simulink model "kurtosis"  (R2012b)
settings: Solver=ode45  StartTime=0.0  StopTime=3171  RelTol=1e-3
libraries: xbsIndex_r4 x3174, casper_library_flow_control x64, casper_library_misc x1, simulink_xsg_bridge x1
(part 2 of 24)

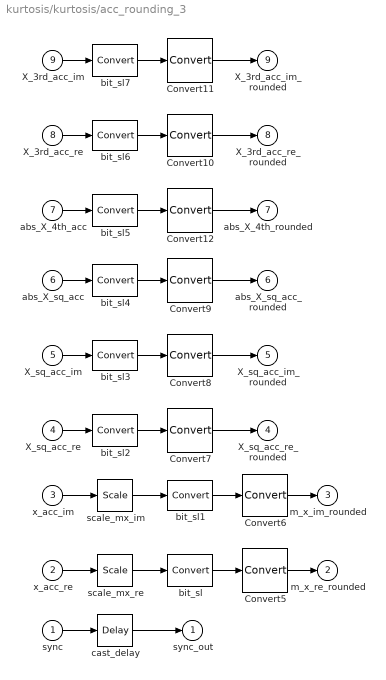
== system kurtosis/kurtosis/acc_rounding_3 ==
  sync : Inport
  x_acc_re : Inport  Port=2
  x_acc_im : Inport  Port=3
  X_sq_acc_re : Inport  Port=4
  X_sq_acc_im : Inport  Port=5
  abs_X_sq_acc : Inport  Port=6
  abs_X_4th_acc : Inport  Port=7
  X_3rd_acc_re : Inport  Port=8
  X_3rd_acc_im : Inport  Port=9
  Convert{7..11} (5 alike) : xbsIndex_r4/Convert  gui_display_data_type=Fixed-point  arith_type="Signed  (2's comp)"  n_bits=35  bin_pt=22  float_type=Single  exp_bits=8  fraction_bits=24  quantization="Round  (unbiased: +/- Inf)"  overflow=Saturate  en=off  latency=5  dbl_ovrd=off  pipeline=off  block_type=convert
  Convert12 : xbsIndex_r4/Convert  gui_display_data_type=Fixed-point  arith_type="Signed  (2's comp)"  n_bits=84  bin_pt=68  float_type=Single  exp_bits=8  fraction_bits=24  quantization="Round  (unbiased: +/- Inf)"  overflow=Saturate  en=off  latency=5  dbl_ovrd=off  pipeline=off  block_type=convert
  Convert5 : xbsIndex_r4/Convert  gui_display_data_type=Fixed-point  arith_type="Signed  (2's comp)"  n_bits=25  bin_pt=24  float_type=Single  exp_bits=8  fraction_bits=24  quantization="Round  (unbiased: +/- Inf)"  overflow=Saturate  en=off  latency=5  dbl_ovrd=off  pipeline=off  block_type=convert
  Convert6 : xbsIndex_r4/Convert  gui_display_data_type=Fixed-point  arith_type="Signed  (2's comp)"  n_bits=25  bin_pt=24  float_type=Single  exp_bits=8  fraction_bits=24  quantization="Round  (unbiased: +/- Inf)"  overflow=Saturate  en=off  latency=5  dbl_ovrd=off  pipeline=off  block_type=convert
  bit_sl : xbsIndex_r4/Convert  gui_display_data_type=Fixed-point  arith_type="Signed  (2's comp)"  n_bits=28  bin_pt=27  float_type=Single  exp_bits=8  fraction_bits=24  quantization=Truncate  overflow=Wrap  en=off  latency=0  dbl_ovrd=off  pipeline=off  block_type=convert
  bit_sl1 : xbsIndex_r4/Convert  gui_display_data_type=Fixed-point  arith_type="Signed  (2's comp)"  n_bits=28  bin_pt=27  float_type=Single  exp_bits=8  fraction_bits=24  quantization=Truncate  overflow=Wrap  en=off  latency=0  dbl_ovrd=off  pipeline=off  block_type=convert
  bit_sl2 : xbsIndex_r4/Convert  gui_display_data_type=Fixed-point  arith_type="Signed  (2's comp)"  n_bits=47  bin_pt=34  float_type=Single  exp_bits=8  fraction_bits=24  quantization=Truncate  overflow=Wrap  en=off  latency=0  dbl_ovrd=off  pipeline=off  block_type=convert
  bit_sl3 : xbsIndex_r4/Convert  gui_display_data_type=Fixed-point  arith_type="Signed  (2's comp)"  n_bits=47  bin_pt=34  float_type=Single  exp_bits=8  fraction_bits=24  quantization=Truncate  overflow=Wrap  en=off  latency=0  dbl_ovrd=off  pipeline=off  block_type=convert
  bit_sl4 : xbsIndex_r4/Convert  gui_display_data_type=Fixed-point  arith_type="Signed  (2's comp)"  n_bits=47  bin_pt=34  float_type=Single  exp_bits=8  fraction_bits=24  quantization=Truncate  overflow=Wrap  en=off  latency=0  dbl_ovrd=off  pipeline=off  block_type=convert
  bit_sl5 : xbsIndex_r4/Convert  gui_display_data_type=Fixed-point  arith_type="Signed  (2's comp)"  n_bits=84  bin_pt=68  float_type=Single  exp_bits=8  fraction_bits=24  quantization=Truncate  overflow=Wrap  en=off  latency=0  dbl_ovrd=off  pipeline=off  block_type=convert
  bit_sl6 : xbsIndex_r4/Convert  gui_display_data_type=Fixed-point  arith_type="Signed  (2's comp)"  n_bits=64  bin_pt=51  float_type=Single  exp_bits=8  fraction_bits=24  quantization=Truncate  overflow=Wrap  en=off  latency=0  dbl_ovrd=off  pipeline=off  block_type=convert
  bit_sl7 : xbsIndex_r4/Convert  gui_display_data_type=Fixed-point  arith_type="Signed  (2's comp)"  n_bits=64  bin_pt=51  float_type=Single  exp_bits=8  fraction_bits=24  quantization=Truncate  overflow=Wrap  en=off  latency=0  dbl_ovrd=off  pipeline=off  block_type=convert
  cast_delay : xbsIndex_r4/Delay  rst=off  infoeditControl=Selection of Reset will increase slice count due to use of real FFs and instead of SRLs  en=off  latency=5  dbl_ovrd=off  reg_retiming=off  block_type=delay
  scale_mx_im : xbsIndex_r4/Scale  scale_factor=-10  dbl_ovrd=off  block_type=scale
  scale_mx_re : xbsIndex_r4/Scale  scale_factor=-10  dbl_ovrd=off  block_type=scale
  sync_out : Outport
  m_x_re_rounded : Outport  Port=2
  m_x_im_rounded : Outport  Port=3
  X_sq_acc_re_rounded : Outport  Port=4
  X_sq_acc_im_rounded : Outport  Port=5
  abs_X_sq_acc_rounded : Outport  Port=6
  abs_X_4th_rounded : Outport  Port=7
  X_3rd_acc_re_rounded : Outport  Port=8
  X_3rd_acc_im_rounded : Outport  Port=9
  wires:
  cast_delay/1 -> sync_out/1
  sync/1 -> cast_delay/1
  Convert11/1 -> X_3rd_acc_im_rounded/1
  bit_sl7/1 -> Convert11/1
  Convert10/1 -> X_3rd_acc_re_rounded/1
  bit_sl6/1 -> Convert10/1
  Convert12/1 -> abs_X_4th_rounded/1
  bit_sl5/1 -> Convert12/1
  Convert9/1 -> abs_X_sq_acc_rounded/1
  bit_sl4/1 -> Convert9/1
  Convert8/1 -> X_sq_acc_im_rounded/1
  bit_sl3/1 -> Convert8/1
  Convert7/1 -> X_sq_acc_re_rounded/1
  bit_sl2/1 -> Convert7/1
  Convert6/1 -> m_x_im_rounded/1
  bit_sl1/1 -> Convert6/1
  Convert5/1 -> m_x_re_rounded/1
  bit_sl/1 -> Convert5/1
  X_3rd_acc_im/1 -> bit_sl7/1
  X_3rd_acc_re/1 -> bit_sl6/1
  abs_X_4th_acc/1 -> bit_sl5/1
  abs_X_sq_acc/1 -> bit_sl4/1
  X_sq_acc_im/1 -> bit_sl3/1
  X_sq_acc_re/1 -> bit_sl2/1
  scale_mx_im/1 -> bit_sl1/1
  scale_mx_re/1 -> bit_sl/1
  x_acc_im/1 -> scale_mx_im/1
  x_acc_re/1 -> scale_mx_re/1

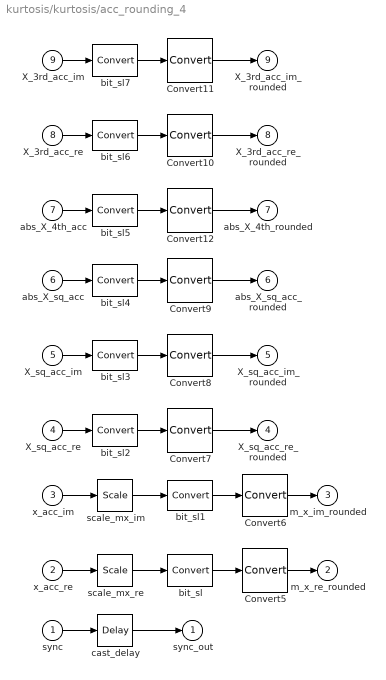
== system kurtosis/kurtosis/acc_rounding_4 ==
  sync : Inport
  x_acc_re : Inport  Port=2
  x_acc_im : Inport  Port=3
  X_sq_acc_re : Inport  Port=4
  X_sq_acc_im : Inport  Port=5
  abs_X_sq_acc : Inport  Port=6
  abs_X_4th_acc : Inport  Port=7
  X_3rd_acc_re : Inport  Port=8
  X_3rd_acc_im : Inport  Port=9
  Convert{7..11} (5 alike) : xbsIndex_r4/Convert  gui_display_data_type=Fixed-point  arith_type="Signed  (2's comp)"  n_bits=35  bin_pt=22  float_type=Single  exp_bits=8  fraction_bits=24  quantization="Round  (unbiased: +/- Inf)"  overflow=Saturate  en=off  latency=5  dbl_ovrd=off  pipeline=off  block_type=convert
  Convert12 : xbsIndex_r4/Convert  gui_display_data_type=Fixed-point  arith_type="Signed  (2's comp)"  n_bits=84  bin_pt=68  float_type=Single  exp_bits=8  fraction_bits=24  quantization="Round  (unbiased: +/- Inf)"  overflow=Saturate  en=off  latency=5  dbl_ovrd=off  pipeline=off  block_type=convert
  Convert5 : xbsIndex_r4/Convert  gui_display_data_type=Fixed-point  arith_type="Signed  (2's comp)"  n_bits=25  bin_pt=24  float_type=Single  exp_bits=8  fraction_bits=24  quantization="Round  (unbiased: +/- Inf)"  overflow=Saturate  en=off  latency=5  dbl_ovrd=off  pipeline=off  block_type=convert
  Convert6 : xbsIndex_r4/Convert  gui_display_data_type=Fixed-point  arith_type="Signed  (2's comp)"  n_bits=25  bin_pt=24  float_type=Single  exp_bits=8  fraction_bits=24  quantization="Round  (unbiased: +/- Inf)"  overflow=Saturate  en=off  latency=5  dbl_ovrd=off  pipeline=off  block_type=convert
  bit_sl : xbsIndex_r4/Convert  gui_display_data_type=Fixed-point  arith_type="Signed  (2's comp)"  n_bits=28  bin_pt=27  float_type=Single  exp_bits=8  fraction_bits=24  quantization=Truncate  overflow=Wrap  en=off  latency=0  dbl_ovrd=off  pipeline=off  block_type=convert
  bit_sl1 : xbsIndex_r4/Convert  gui_display_data_type=Fixed-point  arith_type="Signed  (2's comp)"  n_bits=28  bin_pt=27  float_type=Single  exp_bits=8  fraction_bits=24  quantization=Truncate  overflow=Wrap  en=off  latency=0  dbl_ovrd=off  pipeline=off  block_type=convert
  bit_sl2 : xbsIndex_r4/Convert  gui_display_data_type=Fixed-point  arith_type="Signed  (2's comp)"  n_bits=47  bin_pt=34  float_type=Single  exp_bits=8  fraction_bits=24  quantization=Truncate  overflow=Wrap  en=off  latency=0  dbl_ovrd=off  pipeline=off  block_type=convert
  bit_sl3 : xbsIndex_r4/Convert  gui_display_data_type=Fixed-point  arith_type="Signed  (2's comp)"  n_bits=47  bin_pt=34  float_type=Single  exp_bits=8  fraction_bits=24  quantization=Truncate  overflow=Wrap  en=off  latency=0  dbl_ovrd=off  pipeline=off  block_type=convert
  bit_sl4 : xbsIndex_r4/Convert  gui_display_data_type=Fixed-point  arith_type="Signed  (2's comp)"  n_bits=47  bin_pt=34  float_type=Single  exp_bits=8  fraction_bits=24  quantization=Truncate  overflow=Wrap  en=off  latency=0  dbl_ovrd=off  pipeline=off  block_type=convert
  bit_sl5 : xbsIndex_r4/Convert  gui_display_data_type=Fixed-point  arith_type="Signed  (2's comp)"  n_bits=84  bin_pt=68  float_type=Single  exp_bits=8  fraction_bits=24  quantization=Truncate  overflow=Wrap  en=off  latency=0  dbl_ovrd=off  pipeline=off  block_type=convert
  bit_sl6 : xbsIndex_r4/Convert  gui_display_data_type=Fixed-point  arith_type="Signed  (2's comp)"  n_bits=64  bin_pt=51  float_type=Single  exp_bits=8  fraction_bits=24  quantization=Truncate  overflow=Wrap  en=off  latency=0  dbl_ovrd=off  pipeline=off  block_type=convert
  bit_sl7 : xbsIndex_r4/Convert  gui_display_data_type=Fixed-point  arith_type="Signed  (2's comp)"  n_bits=64  bin_pt=51  float_type=Single  exp_bits=8  fraction_bits=24  quantization=Truncate  overflow=Wrap  en=off  latency=0  dbl_ovrd=off  pipeline=off  block_type=convert
  cast_delay : xbsIndex_r4/Delay  rst=off  infoeditControl=Selection of Reset will increase slice count due to use of real FFs and instead of SRLs  en=off  latency=5  dbl_ovrd=off  reg_retiming=off  block_type=delay
  scale_mx_im : xbsIndex_r4/Scale  scale_factor=-10  dbl_ovrd=off  block_type=scale
  scale_mx_re : xbsIndex_r4/Scale  scale_factor=-10  dbl_ovrd=off  block_type=scale
  sync_out : Outport
  m_x_re_rounded : Outport  Port=2
  m_x_im_rounded : Outport  Port=3
  X_sq_acc_re_rounded : Outport  Port=4
  X_sq_acc_im_rounded : Outport  Port=5
  abs_X_sq_acc_rounded : Outport  Port=6
  abs_X_4th_rounded : Outport  Port=7
  X_3rd_acc_re_rounded : Outport  Port=8
  X_3rd_acc_im_rounded : Outport  Port=9
  wires:
  cast_delay/1 -> sync_out/1
  sync/1 -> cast_delay/1
  Convert11/1 -> X_3rd_acc_im_rounded/1
  bit_sl7/1 -> Convert11/1
  Convert10/1 -> X_3rd_acc_re_rounded/1
  bit_sl6/1 -> Convert10/1
  Convert12/1 -> abs_X_4th_rounded/1
  bit_sl5/1 -> Convert12/1
  Convert9/1 -> abs_X_sq_acc_rounded/1
  bit_sl4/1 -> Convert9/1
  Convert8/1 -> X_sq_acc_im_rounded/1
  bit_sl3/1 -> Convert8/1
  Convert7/1 -> X_sq_acc_re_rounded/1
  bit_sl2/1 -> Convert7/1
  Convert6/1 -> m_x_im_rounded/1
  bit_sl1/1 -> Convert6/1
  Convert5/1 -> m_x_re_rounded/1
  bit_sl/1 -> Convert5/1
  X_3rd_acc_im/1 -> bit_sl7/1
  X_3rd_acc_re/1 -> bit_sl6/1
  abs_X_4th_acc/1 -> bit_sl5/1
  abs_X_sq_acc/1 -> bit_sl4/1
  X_sq_acc_im/1 -> bit_sl3/1
  X_sq_acc_re/1 -> bit_sl2/1
  scale_mx_im/1 -> bit_sl1/1
  scale_mx_re/1 -> bit_sl/1
  x_acc_im/1 -> scale_mx_im/1
  x_acc_re/1 -> scale_mx_re/1

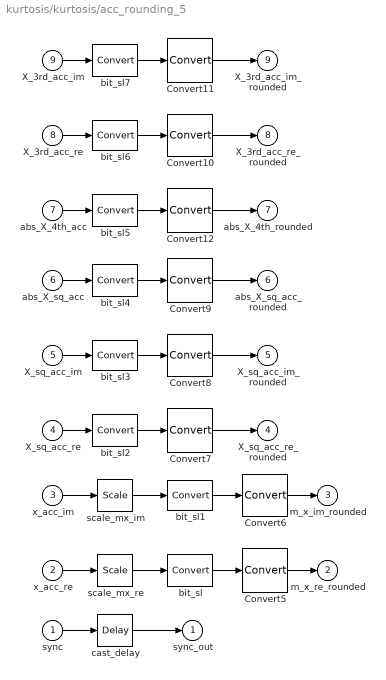
== system kurtosis/kurtosis/acc_rounding_5 ==
  sync : Inport
  x_acc_re : Inport  Port=2
  x_acc_im : Inport  Port=3
  X_sq_acc_re : Inport  Port=4
  X_sq_acc_im : Inport  Port=5
  abs_X_sq_acc : Inport  Port=6
  abs_X_4th_acc : Inport  Port=7
  X_3rd_acc_re : Inport  Port=8
  X_3rd_acc_im : Inport  Port=9
  Convert{7..11} (5 alike) : xbsIndex_r4/Convert  gui_display_data_type=Fixed-point  arith_type="Signed  (2's comp)"  n_bits=35  bin_pt=22  float_type=Single  exp_bits=8  fraction_bits=24  quantization="Round  (unbiased: +/- Inf)"  overflow=Saturate  en=off  latency=5  dbl_ovrd=off  pipeline=off  block_type=convert
  Convert12 : xbsIndex_r4/Convert  gui_display_data_type=Fixed-point  arith_type="Signed  (2's comp)"  n_bits=84  bin_pt=68  float_type=Single  exp_bits=8  fraction_bits=24  quantization="Round  (unbiased: +/- Inf)"  overflow=Saturate  en=off  latency=5  dbl_ovrd=off  pipeline=off  block_type=convert
  Convert5 : xbsIndex_r4/Convert  gui_display_data_type=Fixed-point  arith_type="Signed  (2's comp)"  n_bits=25  bin_pt=24  float_type=Single  exp_bits=8  fraction_bits=24  quantization="Round  (unbiased: +/- Inf)"  overflow=Saturate  en=off  latency=5  dbl_ovrd=off  pipeline=off  block_type=convert
  Convert6 : xbsIndex_r4/Convert  gui_display_data_type=Fixed-point  arith_type="Signed  (2's comp)"  n_bits=25  bin_pt=24  float_type=Single  exp_bits=8  fraction_bits=24  quantization="Round  (unbiased: +/- Inf)"  overflow=Saturate  en=off  latency=5  dbl_ovrd=off  pipeline=off  block_type=convert
  bit_sl : xbsIndex_r4/Convert  gui_display_data_type=Fixed-point  arith_type="Signed  (2's comp)"  n_bits=28  bin_pt=27  float_type=Single  exp_bits=8  fraction_bits=24  quantization=Truncate  overflow=Wrap  en=off  latency=0  dbl_ovrd=off  pipeline=off  block_type=convert
  bit_sl1 : xbsIndex_r4/Convert  gui_display_data_type=Fixed-point  arith_type="Signed  (2's comp)"  n_bits=28  bin_pt=27  float_type=Single  exp_bits=8  fraction_bits=24  quantization=Truncate  overflow=Wrap  en=off  latency=0  dbl_ovrd=off  pipeline=off  block_type=convert
  bit_sl2 : xbsIndex_r4/Convert  gui_display_data_type=Fixed-point  arith_type="Signed  (2's comp)"  n_bits=47  bin_pt=34  float_type=Single  exp_bits=8  fraction_bits=24  quantization=Truncate  overflow=Wrap  en=off  latency=0  dbl_ovrd=off  pipeline=off  block_type=convert
  bit_sl3 : xbsIndex_r4/Convert  gui_display_data_type=Fixed-point  arith_type="Signed  (2's comp)"  n_bits=47  bin_pt=34  float_type=Single  exp_bits=8  fraction_bits=24  quantization=Truncate  overflow=Wrap  en=off  latency=0  dbl_ovrd=off  pipeline=off  block_type=convert
  bit_sl4 : xbsIndex_r4/Convert  gui_display_data_type=Fixed-point  arith_type="Signed  (2's comp)"  n_bits=47  bin_pt=34  float_type=Single  exp_bits=8  fraction_bits=24  quantization=Truncate  overflow=Wrap  en=off  latency=0  dbl_ovrd=off  pipeline=off  block_type=convert
  bit_sl5 : xbsIndex_r4/Convert  gui_display_data_type=Fixed-point  arith_type="Signed  (2's comp)"  n_bits=84  bin_pt=68  float_type=Single  exp_bits=8  fraction_bits=24  quantization=Truncate  overflow=Wrap  en=off  latency=0  dbl_ovrd=off  pipeline=off  block_type=convert
  bit_sl6 : xbsIndex_r4/Convert  gui_display_data_type=Fixed-point  arith_type="Signed  (2's comp)"  n_bits=64  bin_pt=51  float_type=Single  exp_bits=8  fraction_bits=24  quantization=Truncate  overflow=Wrap  en=off  latency=0  dbl_ovrd=off  pipeline=off  block_type=convert
  bit_sl7 : xbsIndex_r4/Convert  gui_display_data_type=Fixed-point  arith_type="Signed  (2's comp)"  n_bits=64  bin_pt=51  float_type=Single  exp_bits=8  fraction_bits=24  quantization=Truncate  overflow=Wrap  en=off  latency=0  dbl_ovrd=off  pipeline=off  block_type=convert
  cast_delay : xbsIndex_r4/Delay  rst=off  infoeditControl=Selection of Reset will increase slice count due to use of real FFs and instead of SRLs  en=off  latency=5  dbl_ovrd=off  reg_retiming=off  block_type=delay
  scale_mx_im : xbsIndex_r4/Scale  scale_factor=-10  dbl_ovrd=off  block_type=scale
  scale_mx_re : xbsIndex_r4/Scale  scale_factor=-10  dbl_ovrd=off  block_type=scale
  sync_out : Outport
  m_x_re_rounded : Outport  Port=2
  m_x_im_rounded : Outport  Port=3
  X_sq_acc_re_rounded : Outport  Port=4
  X_sq_acc_im_rounded : Outport  Port=5
  abs_X_sq_acc_rounded : Outport  Port=6
  abs_X_4th_rounded : Outport  Port=7
  X_3rd_acc_re_rounded : Outport  Port=8
  X_3rd_acc_im_rounded : Outport  Port=9
  wires:
  cast_delay/1 -> sync_out/1
  sync/1 -> cast_delay/1
  Convert11/1 -> X_3rd_acc_im_rounded/1
  bit_sl7/1 -> Convert11/1
  Convert10/1 -> X_3rd_acc_re_rounded/1
  bit_sl6/1 -> Convert10/1
  Convert12/1 -> abs_X_4th_rounded/1
  bit_sl5/1 -> Convert12/1
  Convert9/1 -> abs_X_sq_acc_rounded/1
  bit_sl4/1 -> Convert9/1
  Convert8/1 -> X_sq_acc_im_rounded/1
  bit_sl3/1 -> Convert8/1
  Convert7/1 -> X_sq_acc_re_rounded/1
  bit_sl2/1 -> Convert7/1
  Convert6/1 -> m_x_im_rounded/1
  bit_sl1/1 -> Convert6/1
  Convert5/1 -> m_x_re_rounded/1
  bit_sl/1 -> Convert5/1
  X_3rd_acc_im/1 -> bit_sl7/1
  X_3rd_acc_re/1 -> bit_sl6/1
  abs_X_4th_acc/1 -> bit_sl5/1
  abs_X_sq_acc/1 -> bit_sl4/1
  X_sq_acc_im/1 -> bit_sl3/1
  X_sq_acc_re/1 -> bit_sl2/1
  scale_mx_im/1 -> bit_sl1/1
  scale_mx_re/1 -> bit_sl/1
  x_acc_im/1 -> scale_mx_im/1
  x_acc_re/1 -> scale_mx_re/1

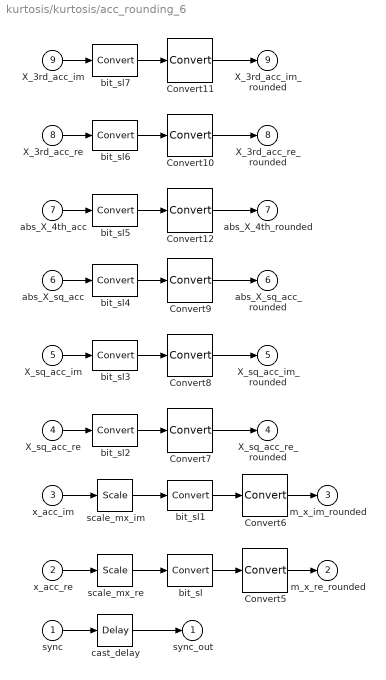
== system kurtosis/kurtosis/acc_rounding_6 ==
  sync : Inport
  x_acc_re : Inport  Port=2
  x_acc_im : Inport  Port=3
  X_sq_acc_re : Inport  Port=4
  X_sq_acc_im : Inport  Port=5
  abs_X_sq_acc : Inport  Port=6
  abs_X_4th_acc : Inport  Port=7
  X_3rd_acc_re : Inport  Port=8
  X_3rd_acc_im : Inport  Port=9
  Convert{7..11} (5 alike) : xbsIndex_r4/Convert  gui_display_data_type=Fixed-point  arith_type="Signed  (2's comp)"  n_bits=35  bin_pt=22  float_type=Single  exp_bits=8  fraction_bits=24  quantization="Round  (unbiased: +/- Inf)"  overflow=Saturate  en=off  latency=5  dbl_ovrd=off  pipeline=off  block_type=convert
  Convert12 : xbsIndex_r4/Convert  gui_display_data_type=Fixed-point  arith_type="Signed  (2's comp)"  n_bits=84  bin_pt=68  float_type=Single  exp_bits=8  fraction_bits=24  quantization="Round  (unbiased: +/- Inf)"  overflow=Saturate  en=off  latency=5  dbl_ovrd=off  pipeline=off  block_type=convert
  Convert5 : xbsIndex_r4/Convert  gui_display_data_type=Fixed-point  arith_type="Signed  (2's comp)"  n_bits=25  bin_pt=24  float_type=Single  exp_bits=8  fraction_bits=24  quantization="Round  (unbiased: +/- Inf)"  overflow=Saturate  en=off  latency=5  dbl_ovrd=off  pipeline=off  block_type=convert
  Convert6 : xbsIndex_r4/Convert  gui_display_data_type=Fixed-point  arith_type="Signed  (2's comp)"  n_bits=25  bin_pt=24  float_type=Single  exp_bits=8  fraction_bits=24  quantization="Round  (unbiased: +/- Inf)"  overflow=Saturate  en=off  latency=5  dbl_ovrd=off  pipeline=off  block_type=convert
  bit_sl : xbsIndex_r4/Convert  gui_display_data_type=Fixed-point  arith_type="Signed  (2's comp)"  n_bits=28  bin_pt=27  float_type=Single  exp_bits=8  fraction_bits=24  quantization=Truncate  overflow=Wrap  en=off  latency=0  dbl_ovrd=off  pipeline=off  block_type=convert
  bit_sl1 : xbsIndex_r4/Convert  gui_display_data_type=Fixed-point  arith_type="Signed  (2's comp)"  n_bits=28  bin_pt=27  float_type=Single  exp_bits=8  fraction_bits=24  quantization=Truncate  overflow=Wrap  en=off  latency=0  dbl_ovrd=off  pipeline=off  block_type=convert
  bit_sl2 : xbsIndex_r4/Convert  gui_display_data_type=Fixed-point  arith_type="Signed  (2's comp)"  n_bits=47  bin_pt=34  float_type=Single  exp_bits=8  fraction_bits=24  quantization=Truncate  overflow=Wrap  en=off  latency=0  dbl_ovrd=off  pipeline=off  block_type=convert
  bit_sl3 : xbsIndex_r4/Convert  gui_display_data_type=Fixed-point  arith_type="Signed  (2's comp)"  n_bits=47  bin_pt=34  float_type=Single  exp_bits=8  fraction_bits=24  quantization=Truncate  overflow=Wrap  en=off  latency=0  dbl_ovrd=off  pipeline=off  block_type=convert
  bit_sl4 : xbsIndex_r4/Convert  gui_display_data_type=Fixed-point  arith_type="Signed  (2's comp)"  n_bits=47  bin_pt=34  float_type=Single  exp_bits=8  fraction_bits=24  quantization=Truncate  overflow=Wrap  en=off  latency=0  dbl_ovrd=off  pipeline=off  block_type=convert
  bit_sl5 : xbsIndex_r4/Convert  gui_display_data_type=Fixed-point  arith_type="Signed  (2's comp)"  n_bits=84  bin_pt=68  float_type=Single  exp_bits=8  fraction_bits=24  quantization=Truncate  overflow=Wrap  en=off  latency=0  dbl_ovrd=off  pipeline=off  block_type=convert
  bit_sl6 : xbsIndex_r4/Convert  gui_display_data_type=Fixed-point  arith_type="Signed  (2's comp)"  n_bits=64  bin_pt=51  float_type=Single  exp_bits=8  fraction_bits=24  quantization=Truncate  overflow=Wrap  en=off  latency=0  dbl_ovrd=off  pipeline=off  block_type=convert
  bit_sl7 : xbsIndex_r4/Convert  gui_display_data_type=Fixed-point  arith_type="Signed  (2's comp)"  n_bits=64  bin_pt=51  float_type=Single  exp_bits=8  fraction_bits=24  quantization=Truncate  overflow=Wrap  en=off  latency=0  dbl_ovrd=off  pipeline=off  block_type=convert
  cast_delay : xbsIndex_r4/Delay  rst=off  infoeditControl=Selection of Reset will increase slice count due to use of real FFs and instead of SRLs  en=off  latency=5  dbl_ovrd=off  reg_retiming=off  block_type=delay
  scale_mx_im : xbsIndex_r4/Scale  scale_factor=-10  dbl_ovrd=off  block_type=scale
  scale_mx_re : xbsIndex_r4/Scale  scale_factor=-10  dbl_ovrd=off  block_type=scale
  sync_out : Outport
  m_x_re_rounded : Outport  Port=2
  m_x_im_rounded : Outport  Port=3
  X_sq_acc_re_rounded : Outport  Port=4
  X_sq_acc_im_rounded : Outport  Port=5
  abs_X_sq_acc_rounded : Outport  Port=6
  abs_X_4th_rounded : Outport  Port=7
  X_3rd_acc_re_rounded : Outport  Port=8
  X_3rd_acc_im_rounded : Outport  Port=9
  wires:
  cast_delay/1 -> sync_out/1
  sync/1 -> cast_delay/1
  Convert11/1 -> X_3rd_acc_im_rounded/1
  bit_sl7/1 -> Convert11/1
  Convert10/1 -> X_3rd_acc_re_rounded/1
  bit_sl6/1 -> Convert10/1
  Convert12/1 -> abs_X_4th_rounded/1
  bit_sl5/1 -> Convert12/1
  Convert9/1 -> abs_X_sq_acc_rounded/1
  bit_sl4/1 -> Convert9/1
  Convert8/1 -> X_sq_acc_im_rounded/1
  bit_sl3/1 -> Convert8/1
  Convert7/1 -> X_sq_acc_re_rounded/1
  bit_sl2/1 -> Convert7/1
  Convert6/1 -> m_x_im_rounded/1
  bit_sl1/1 -> Convert6/1
  Convert5/1 -> m_x_re_rounded/1
  bit_sl/1 -> Convert5/1
  X_3rd_acc_im/1 -> bit_sl7/1
  X_3rd_acc_re/1 -> bit_sl6/1
  abs_X_4th_acc/1 -> bit_sl5/1
  abs_X_sq_acc/1 -> bit_sl4/1
  X_sq_acc_im/1 -> bit_sl3/1
  X_sq_acc_re/1 -> bit_sl2/1
  scale_mx_im/1 -> bit_sl1/1
  scale_mx_re/1 -> bit_sl/1
  x_acc_im/1 -> scale_mx_im/1
  x_acc_re/1 -> scale_mx_re/1

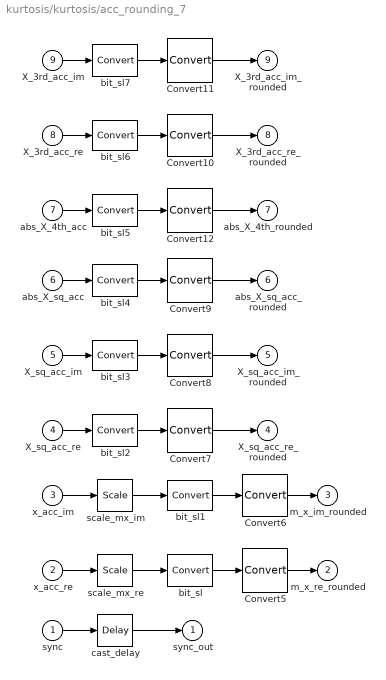
== system kurtosis/kurtosis/acc_rounding_7 ==
  sync : Inport
  x_acc_re : Inport  Port=2
  x_acc_im : Inport  Port=3
  X_sq_acc_re : Inport  Port=4
  X_sq_acc_im : Inport  Port=5
  abs_X_sq_acc : Inport  Port=6
  abs_X_4th_acc : Inport  Port=7
  X_3rd_acc_re : Inport  Port=8
  X_3rd_acc_im : Inport  Port=9
  Convert{7..11} (5 alike) : xbsIndex_r4/Convert  gui_display_data_type=Fixed-point  arith_type="Signed  (2's comp)"  n_bits=35  bin_pt=22  float_type=Single  exp_bits=8  fraction_bits=24  quantization="Round  (unbiased: +/- Inf)"  overflow=Saturate  en=off  latency=5  dbl_ovrd=off  pipeline=off  block_type=convert
  Convert12 : xbsIndex_r4/Convert  gui_display_data_type=Fixed-point  arith_type="Signed  (2's comp)"  n_bits=84  bin_pt=68  float_type=Single  exp_bits=8  fraction_bits=24  quantization="Round  (unbiased: +/- Inf)"  overflow=Saturate  en=off  latency=5  dbl_ovrd=off  pipeline=off  block_type=convert
  Convert5 : xbsIndex_r4/Convert  gui_display_data_type=Fixed-point  arith_type="Signed  (2's comp)"  n_bits=25  bin_pt=24  float_type=Single  exp_bits=8  fraction_bits=24  quantization="Round  (unbiased: +/- Inf)"  overflow=Saturate  en=off  latency=5  dbl_ovrd=off  pipeline=off  block_type=convert
  Convert6 : xbsIndex_r4/Convert  gui_display_data_type=Fixed-point  arith_type="Signed  (2's comp)"  n_bits=25  bin_pt=24  float_type=Single  exp_bits=8  fraction_bits=24  quantization="Round  (unbiased: +/- Inf)"  overflow=Saturate  en=off  latency=5  dbl_ovrd=off  pipeline=off  block_type=convert
  bit_sl : xbsIndex_r4/Convert  gui_display_data_type=Fixed-point  arith_type="Signed  (2's comp)"  n_bits=28  bin_pt=27  float_type=Single  exp_bits=8  fraction_bits=24  quantization=Truncate  overflow=Wrap  en=off  latency=0  dbl_ovrd=off  pipeline=off  block_type=convert
  bit_sl1 : xbsIndex_r4/Convert  gui_display_data_type=Fixed-point  arith_type="Signed  (2's comp)"  n_bits=28  bin_pt=27  float_type=Single  exp_bits=8  fraction_bits=24  quantization=Truncate  overflow=Wrap  en=off  latency=0  dbl_ovrd=off  pipeline=off  block_type=convert
  bit_sl2 : xbsIndex_r4/Convert  gui_display_data_type=Fixed-point  arith_type="Signed  (2's comp)"  n_bits=47  bin_pt=34  float_type=Single  exp_bits=8  fraction_bits=24  quantization=Truncate  overflow=Wrap  en=off  latency=0  dbl_ovrd=off  pipeline=off  block_type=convert
  bit_sl3 : xbsIndex_r4/Convert  gui_display_data_type=Fixed-point  arith_type="Signed  (2's comp)"  n_bits=47  bin_pt=34  float_type=Single  exp_bits=8  fraction_bits=24  quantization=Truncate  overflow=Wrap  en=off  latency=0  dbl_ovrd=off  pipeline=off  block_type=convert
  bit_sl4 : xbsIndex_r4/Convert  gui_display_data_type=Fixed-point  arith_type="Signed  (2's comp)"  n_bits=47  bin_pt=34  float_type=Single  exp_bits=8  fraction_bits=24  quantization=Truncate  overflow=Wrap  en=off  latency=0  dbl_ovrd=off  pipeline=off  block_type=convert
  bit_sl5 : xbsIndex_r4/Convert  gui_display_data_type=Fixed-point  arith_type="Signed  (2's comp)"  n_bits=84  bin_pt=68  float_type=Single  exp_bits=8  fraction_bits=24  quantization=Truncate  overflow=Wrap  en=off  latency=0  dbl_ovrd=off  pipeline=off  block_type=convert
  bit_sl6 : xbsIndex_r4/Convert  gui_display_data_type=Fixed-point  arith_type="Signed  (2's comp)"  n_bits=64  bin_pt=51  float_type=Single  exp_bits=8  fraction_bits=24  quantization=Truncate  overflow=Wrap  en=off  latency=0  dbl_ovrd=off  pipeline=off  block_type=convert
  bit_sl7 : xbsIndex_r4/Convert  gui_display_data_type=Fixed-point  arith_type="Signed  (2's comp)"  n_bits=64  bin_pt=51  float_type=Single  exp_bits=8  fraction_bits=24  quantization=Truncate  overflow=Wrap  en=off  latency=0  dbl_ovrd=off  pipeline=off  block_type=convert
  cast_delay : xbsIndex_r4/Delay  rst=off  infoeditControl=Selection of Reset will increase slice count due to use of real FFs and instead of SRLs  en=off  latency=5  dbl_ovrd=off  reg_retiming=off  block_type=delay
  scale_mx_im : xbsIndex_r4/Scale  scale_factor=-10  dbl_ovrd=off  block_type=scale
  scale_mx_re : xbsIndex_r4/Scale  scale_factor=-10  dbl_ovrd=off  block_type=scale
  sync_out : Outport
  m_x_re_rounded : Outport  Port=2
  m_x_im_rounded : Outport  Port=3
  X_sq_acc_re_rounded : Outport  Port=4
  X_sq_acc_im_rounded : Outport  Port=5
  abs_X_sq_acc_rounded : Outport  Port=6
  abs_X_4th_rounded : Outport  Port=7
  X_3rd_acc_re_rounded : Outport  Port=8
  X_3rd_acc_im_rounded : Outport  Port=9
  wires:
  cast_delay/1 -> sync_out/1
  sync/1 -> cast_delay/1
  Convert11/1 -> X_3rd_acc_im_rounded/1
  bit_sl7/1 -> Convert11/1
  Convert10/1 -> X_3rd_acc_re_rounded/1
  bit_sl6/1 -> Convert10/1
  Convert12/1 -> abs_X_4th_rounded/1
  bit_sl5/1 -> Convert12/1
  Convert9/1 -> abs_X_sq_acc_rounded/1
  bit_sl4/1 -> Convert9/1
  Convert8/1 -> X_sq_acc_im_rounded/1
  bit_sl3/1 -> Convert8/1
  Convert7/1 -> X_sq_acc_re_rounded/1
  bit_sl2/1 -> Convert7/1
  Convert6/1 -> m_x_im_rounded/1
  bit_sl1/1 -> Convert6/1
  Convert5/1 -> m_x_re_rounded/1
  bit_sl/1 -> Convert5/1
  X_3rd_acc_im/1 -> bit_sl7/1
  X_3rd_acc_re/1 -> bit_sl6/1
  abs_X_4th_acc/1 -> bit_sl5/1
  abs_X_sq_acc/1 -> bit_sl4/1
  X_sq_acc_im/1 -> bit_sl3/1
  X_sq_acc_re/1 -> bit_sl2/1
  scale_mx_im/1 -> bit_sl1/1
  scale_mx_re/1 -> bit_sl/1
  x_acc_im/1 -> scale_mx_im/1
  x_acc_re/1 -> scale_mx_re/1

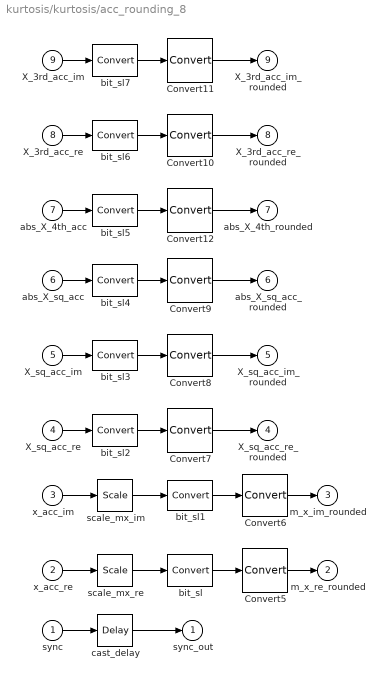
== system kurtosis/kurtosis/acc_rounding_8 ==
  sync : Inport
  x_acc_re : Inport  Port=2
  x_acc_im : Inport  Port=3
  X_sq_acc_re : Inport  Port=4
  X_sq_acc_im : Inport  Port=5
  abs_X_sq_acc : Inport  Port=6
  abs_X_4th_acc : Inport  Port=7
  X_3rd_acc_re : Inport  Port=8
  X_3rd_acc_im : Inport  Port=9
  Convert{7..11} (5 alike) : xbsIndex_r4/Convert  gui_display_data_type=Fixed-point  arith_type="Signed  (2's comp)"  n_bits=35  bin_pt=22  float_type=Single  exp_bits=8  fraction_bits=24  quantization="Round  (unbiased: +/- Inf)"  overflow=Saturate  en=off  latency=5  dbl_ovrd=off  pipeline=off  block_type=convert
  Convert12 : xbsIndex_r4/Convert  gui_display_data_type=Fixed-point  arith_type="Signed  (2's comp)"  n_bits=84  bin_pt=68  float_type=Single  exp_bits=8  fraction_bits=24  quantization="Round  (unbiased: +/- Inf)"  overflow=Saturate  en=off  latency=5  dbl_ovrd=off  pipeline=off  block_type=convert
  Convert5 : xbsIndex_r4/Convert  gui_display_data_type=Fixed-point  arith_type="Signed  (2's comp)"  n_bits=25  bin_pt=24  float_type=Single  exp_bits=8  fraction_bits=24  quantization="Round  (unbiased: +/- Inf)"  overflow=Saturate  en=off  latency=5  dbl_ovrd=off  pipeline=off  block_type=convert
  Convert6 : xbsIndex_r4/Convert  gui_display_data_type=Fixed-point  arith_type="Signed  (2's comp)"  n_bits=25  bin_pt=24  float_type=Single  exp_bits=8  fraction_bits=24  quantization="Round  (unbiased: +/- Inf)"  overflow=Saturate  en=off  latency=5  dbl_ovrd=off  pipeline=off  block_type=convert
  bit_sl : xbsIndex_r4/Convert  gui_display_data_type=Fixed-point  arith_type="Signed  (2's comp)"  n_bits=28  bin_pt=27  float_type=Single  exp_bits=8  fraction_bits=24  quantization=Truncate  overflow=Wrap  en=off  latency=0  dbl_ovrd=off  pipeline=off  block_type=convert
  bit_sl1 : xbsIndex_r4/Convert  gui_display_data_type=Fixed-point  arith_type="Signed  (2's comp)"  n_bits=28  bin_pt=27  float_type=Single  exp_bits=8  fraction_bits=24  quantization=Truncate  overflow=Wrap  en=off  latency=0  dbl_ovrd=off  pipeline=off  block_type=convert
  bit_sl2 : xbsIndex_r4/Convert  gui_display_data_type=Fixed-point  arith_type="Signed  (2's comp)"  n_bits=47  bin_pt=34  float_type=Single  exp_bits=8  fraction_bits=24  quantization=Truncate  overflow=Wrap  en=off  latency=0  dbl_ovrd=off  pipeline=off  block_type=convert
  bit_sl3 : xbsIndex_r4/Convert  gui_display_data_type=Fixed-point  arith_type="Signed  (2's comp)"  n_bits=47  bin_pt=34  float_type=Single  exp_bits=8  fraction_bits=24  quantization=Truncate  overflow=Wrap  en=off  latency=0  dbl_ovrd=off  pipeline=off  block_type=convert
  bit_sl4 : xbsIndex_r4/Convert  gui_display_data_type=Fixed-point  arith_type="Signed  (2's comp)"  n_bits=47  bin_pt=34  float_type=Single  exp_bits=8  fraction_bits=24  quantization=Truncate  overflow=Wrap  en=off  latency=0  dbl_ovrd=off  pipeline=off  block_type=convert
  bit_sl5 : xbsIndex_r4/Convert  gui_display_data_type=Fixed-point  arith_type="Signed  (2's comp)"  n_bits=84  bin_pt=68  float_type=Single  exp_bits=8  fraction_bits=24  quantization=Truncate  overflow=Wrap  en=off  latency=0  dbl_ovrd=off  pipeline=off  block_type=convert
  bit_sl6 : xbsIndex_r4/Convert  gui_display_data_type=Fixed-point  arith_type="Signed  (2's comp)"  n_bits=64  bin_pt=51  float_type=Single  exp_bits=8  fraction_bits=24  quantization=Truncate  overflow=Wrap  en=off  latency=0  dbl_ovrd=off  pipeline=off  block_type=convert
  bit_sl7 : xbsIndex_r4/Convert  gui_display_data_type=Fixed-point  arith_type="Signed  (2's comp)"  n_bits=64  bin_pt=51  float_type=Single  exp_bits=8  fraction_bits=24  quantization=Truncate  overflow=Wrap  en=off  latency=0  dbl_ovrd=off  pipeline=off  block_type=convert
  cast_delay : xbsIndex_r4/Delay  rst=off  infoeditControl=Selection of Reset will increase slice count due to use of real FFs and instead of SRLs  en=off  latency=5  dbl_ovrd=off  reg_retiming=off  block_type=delay
  scale_mx_im : xbsIndex_r4/Scale  scale_factor=-10  dbl_ovrd=off  block_type=scale
  scale_mx_re : xbsIndex_r4/Scale  scale_factor=-10  dbl_ovrd=off  block_type=scale
  sync_out : Outport
  m_x_re_rounded : Outport  Port=2
  m_x_im_rounded : Outport  Port=3
  X_sq_acc_re_rounded : Outport  Port=4
  X_sq_acc_im_rounded : Outport  Port=5
  abs_X_sq_acc_rounded : Outport  Port=6
  abs_X_4th_rounded : Outport  Port=7
  X_3rd_acc_re_rounded : Outport  Port=8
  X_3rd_acc_im_rounded : Outport  Port=9
  wires:
  cast_delay/1 -> sync_out/1
  sync/1 -> cast_delay/1
  Convert11/1 -> X_3rd_acc_im_rounded/1
  bit_sl7/1 -> Convert11/1
  Convert10/1 -> X_3rd_acc_re_rounded/1
  bit_sl6/1 -> Convert10/1
  Convert12/1 -> abs_X_4th_rounded/1
  bit_sl5/1 -> Convert12/1
  Convert9/1 -> abs_X_sq_acc_rounded/1
  bit_sl4/1 -> Convert9/1
  Convert8/1 -> X_sq_acc_im_rounded/1
  bit_sl3/1 -> Convert8/1
  Convert7/1 -> X_sq_acc_re_rounded/1
  bit_sl2/1 -> Convert7/1
  Convert6/1 -> m_x_im_rounded/1
  bit_sl1/1 -> Convert6/1
  Convert5/1 -> m_x_re_rounded/1
  bit_sl/1 -> Convert5/1
  X_3rd_acc_im/1 -> bit_sl7/1
  X_3rd_acc_re/1 -> bit_sl6/1
  abs_X_4th_acc/1 -> bit_sl5/1
  abs_X_sq_acc/1 -> bit_sl4/1
  X_sq_acc_im/1 -> bit_sl3/1
  X_sq_acc_re/1 -> bit_sl2/1
  scale_mx_im/1 -> bit_sl1/1
  scale_mx_re/1 -> bit_sl/1
  x_acc_im/1 -> scale_mx_im/1
  x_acc_re/1 -> scale_mx_re/1

== system kurtosis/kurtosis/kurtosis_acc_bank_1 ==
  sync : Inport
  x : Inport  Port=2
  x^2 : Inport  Port=3
  |x|^2 : Inport  Port=4
  |x|^4 : Inport  Port=5
  x|x|^2 : Inport  Port=6
  abs_x_4th_acc : Subsystem
  abs_x_sq_acc : Subsystem
  acc_rst : Subsystem
  x_acc : Subsystem
  x_cube_acc : Subsystem
  x_sq_acc : Subsystem
  sync_out : Outport
  "Re{E[x]}" : Outport  Port=2
  "Im{E[x]}" : Outport  Port=3
  "Re{E[x^2]}" : Outport  Port=4
  "Im{E[x^2]}" : Outport  Port=5
  E[|x|^2] : Outport  Port=6
  E[|x|^4] : Outport  Port=7
  "Re{E[x|x|^2]}" : Outport  Port=8
  "Im{E[x|x|^2]}" : Outport  Port=9
  wires:
  acc_rst/1(acc_rst) -> abs_x_4th_acc/1(sync), abs_x_sq_acc/1(sync), x_cube_acc/1(sync), x_sq_acc/1(sync), x_acc/1(sync)  "acc_rst"
  abs_x_4th_acc/1(+=b) -> E[|x|^4]/1
  |x|^4/1 -> abs_x_4th_acc/2(b)
  abs_x_sq_acc/1(+=b) -> E[|x|^2]/1
  |x|^2/1 -> abs_x_sq_acc/2(b)
  x_cube_acc/2(x_im_acc) -> "Im{E[x|x|^2]}"/1
  x_cube_acc/1(x_re_acc) -> "Re{E[x|x|^2]}"/1
  x|x|^2/1 -> x_cube_acc/2(x)
  x_sq_acc/2(x_im_acc) -> "Im{E[x^2]}"/1
  x_sq_acc/1(x_re_acc) -> "Re{E[x^2]}"/1
  x^2/1 -> x_sq_acc/2(x)
  x_acc/2(x_im_acc) -> "Im{E[x]}"/1
  x_acc/1(x_re_acc) -> "Re{E[x]}"/1
  x/1 -> x_acc/2(x)
  acc_rst/2(sync_out) -> sync_out/1
  sync/1 -> acc_rst/1(sync)

== system kurtosis/kurtosis/kurtosis_acc_bank_2 ==
  sync : Inport
  x : Inport  Port=2
  x^2 : Inport  Port=3
  |x|^2 : Inport  Port=4
  |x|^4 : Inport  Port=5
  x|x|^2 : Inport  Port=6
  abs_x_4th_acc : Subsystem
  abs_x_sq_acc : Subsystem
  acc_rst : Subsystem
  x_acc : Subsystem
  x_cube_acc : Subsystem
  x_sq_acc : Subsystem
  sync_out : Outport
  "Re{E[x]}" : Outport  Port=2
  "Im{E[x]}" : Outport  Port=3
  "Re{E[x^2]}" : Outport  Port=4
  "Im{E[x^2]}" : Outport  Port=5
  E[|x|^2] : Outport  Port=6
  E[|x|^4] : Outport  Port=7
  "Re{E[x|x|^2]}" : Outport  Port=8
  "Im{E[x|x|^2]}" : Outport  Port=9
  wires:
  acc_rst/1(acc_rst) -> abs_x_4th_acc/1(sync), abs_x_sq_acc/1(sync), x_cube_acc/1(sync), x_sq_acc/1(sync), x_acc/1(sync)  "acc_rst"
  abs_x_4th_acc/1(+=b) -> E[|x|^4]/1
  |x|^4/1 -> abs_x_4th_acc/2(b)
  abs_x_sq_acc/1(+=b) -> E[|x|^2]/1
  |x|^2/1 -> abs_x_sq_acc/2(b)
  x_cube_acc/2(x_im_acc) -> "Im{E[x|x|^2]}"/1
  x_cube_acc/1(x_re_acc) -> "Re{E[x|x|^2]}"/1
  x|x|^2/1 -> x_cube_acc/2(x)
  x_sq_acc/2(x_im_acc) -> "Im{E[x^2]}"/1
  x_sq_acc/1(x_re_acc) -> "Re{E[x^2]}"/1
  x^2/1 -> x_sq_acc/2(x)
  x_acc/2(x_im_acc) -> "Im{E[x]}"/1
  x_acc/1(x_re_acc) -> "Re{E[x]}"/1
  x/1 -> x_acc/2(x)
  acc_rst/2(sync_out) -> sync_out/1
  sync/1 -> acc_rst/1(sync)

== system kurtosis/kurtosis/kurtosis_acc_bank_3 ==
  sync : Inport
  x : Inport  Port=2
  x^2 : Inport  Port=3
  |x|^2 : Inport  Port=4
  |x|^4 : Inport  Port=5
  x|x|^2 : Inport  Port=6
  abs_x_4th_acc : Subsystem
  abs_x_sq_acc : Subsystem
  acc_rst : Subsystem
  x_acc : Subsystem
  x_cube_acc : Subsystem
  x_sq_acc : Subsystem
  sync_out : Outport
  "Re{E[x]}" : Outport  Port=2
  "Im{E[x]}" : Outport  Port=3
  "Re{E[x^2]}" : Outport  Port=4
  "Im{E[x^2]}" : Outport  Port=5
  E[|x|^2] : Outport  Port=6
  E[|x|^4] : Outport  Port=7
  "Re{E[x|x|^2]}" : Outport  Port=8
  "Im{E[x|x|^2]}" : Outport  Port=9
  wires:
  acc_rst/1(acc_rst) -> abs_x_4th_acc/1(sync), abs_x_sq_acc/1(sync), x_cube_acc/1(sync), x_sq_acc/1(sync), x_acc/1(sync)  "acc_rst"
  abs_x_4th_acc/1(+=b) -> E[|x|^4]/1
  |x|^4/1 -> abs_x_4th_acc/2(b)
  abs_x_sq_acc/1(+=b) -> E[|x|^2]/1
  |x|^2/1 -> abs_x_sq_acc/2(b)
  x_cube_acc/2(x_im_acc) -> "Im{E[x|x|^2]}"/1
  x_cube_acc/1(x_re_acc) -> "Re{E[x|x|^2]}"/1
  x|x|^2/1 -> x_cube_acc/2(x)
  x_sq_acc/2(x_im_acc) -> "Im{E[x^2]}"/1
  x_sq_acc/1(x_re_acc) -> "Re{E[x^2]}"/1
  x^2/1 -> x_sq_acc/2(x)
  x_acc/2(x_im_acc) -> "Im{E[x]}"/1
  x_acc/1(x_re_acc) -> "Re{E[x]}"/1
  x/1 -> x_acc/2(x)
  acc_rst/2(sync_out) -> sync_out/1
  sync/1 -> acc_rst/1(sync)

== system kurtosis/kurtosis/kurtosis_acc_bank_4 ==
  sync : Inport
  x : Inport  Port=2
  x^2 : Inport  Port=3
  |x|^2 : Inport  Port=4
  |x|^4 : Inport  Port=5
  x|x|^2 : Inport  Port=6
  abs_x_4th_acc : Subsystem
  abs_x_sq_acc : Subsystem
  acc_rst : Subsystem
  x_acc : Subsystem
  x_cube_acc : Subsystem
  x_sq_acc : Subsystem
  sync_out : Outport
  "Re{E[x]}" : Outport  Port=2
  "Im{E[x]}" : Outport  Port=3
  "Re{E[x^2]}" : Outport  Port=4
  "Im{E[x^2]}" : Outport  Port=5
  E[|x|^2] : Outport  Port=6
  E[|x|^4] : Outport  Port=7
  "Re{E[x|x|^2]}" : Outport  Port=8
  "Im{E[x|x|^2]}" : Outport  Port=9
  wires:
  acc_rst/1(acc_rst) -> abs_x_4th_acc/1(sync), abs_x_sq_acc/1(sync), x_cube_acc/1(sync), x_sq_acc/1(sync), x_acc/1(sync)  "acc_rst"
  abs_x_4th_acc/1(+=b) -> E[|x|^4]/1
  |x|^4/1 -> abs_x_4th_acc/2(b)
  abs_x_sq_acc/1(+=b) -> E[|x|^2]/1
  |x|^2/1 -> abs_x_sq_acc/2(b)
  x_cube_acc/2(x_im_acc) -> "Im{E[x|x|^2]}"/1
  x_cube_acc/1(x_re_acc) -> "Re{E[x|x|^2]}"/1
  x|x|^2/1 -> x_cube_acc/2(x)
  x_sq_acc/2(x_im_acc) -> "Im{E[x^2]}"/1
  x_sq_acc/1(x_re_acc) -> "Re{E[x^2]}"/1
  x^2/1 -> x_sq_acc/2(x)
  x_acc/2(x_im_acc) -> "Im{E[x]}"/1
  x_acc/1(x_re_acc) -> "Re{E[x]}"/1
  x/1 -> x_acc/2(x)
  acc_rst/2(sync_out) -> sync_out/1
  sync/1 -> acc_rst/1(sync)

== system kurtosis/kurtosis/kurtosis_acc_bank_5 ==
  sync : Inport
  x : Inport  Port=2
  x^2 : Inport  Port=3
  |x|^2 : Inport  Port=4
  |x|^4 : Inport  Port=5
  x|x|^2 : Inport  Port=6
  abs_x_4th_acc : Subsystem
  abs_x_sq_acc : Subsystem
  acc_rst : Subsystem
  x_acc : Subsystem
  x_cube_acc : Subsystem
  x_sq_acc : Subsystem
  sync_out : Outport
  "Re{E[x]}" : Outport  Port=2
  "Im{E[x]}" : Outport  Port=3
  "Re{E[x^2]}" : Outport  Port=4
  "Im{E[x^2]}" : Outport  Port=5
  E[|x|^2] : Outport  Port=6
  E[|x|^4] : Outport  Port=7
  "Re{E[x|x|^2]}" : Outport  Port=8
  "Im{E[x|x|^2]}" : Outport  Port=9
  wires:
  acc_rst/1(acc_rst) -> abs_x_4th_acc/1(sync), abs_x_sq_acc/1(sync), x_cube_acc/1(sync), x_sq_acc/1(sync), x_acc/1(sync)  "acc_rst"
  abs_x_4th_acc/1(+=b) -> E[|x|^4]/1
  |x|^4/1 -> abs_x_4th_acc/2(b)
  abs_x_sq_acc/1(+=b) -> E[|x|^2]/1
  |x|^2/1 -> abs_x_sq_acc/2(b)
  x_cube_acc/2(x_im_acc) -> "Im{E[x|x|^2]}"/1
  x_cube_acc/1(x_re_acc) -> "Re{E[x|x|^2]}"/1
  x|x|^2/1 -> x_cube_acc/2(x)
  x_sq_acc/2(x_im_acc) -> "Im{E[x^2]}"/1
  x_sq_acc/1(x_re_acc) -> "Re{E[x^2]}"/1
  x^2/1 -> x_sq_acc/2(x)
  x_acc/2(x_im_acc) -> "Im{E[x]}"/1
  x_acc/1(x_re_acc) -> "Re{E[x]}"/1
  x/1 -> x_acc/2(x)
  acc_rst/2(sync_out) -> sync_out/1
  sync/1 -> acc_rst/1(sync)

== system kurtosis/kurtosis/kurtosis_acc_bank_6 ==
  sync : Inport
  x : Inport  Port=2
  x^2 : Inport  Port=3
  |x|^2 : Inport  Port=4
  |x|^4 : Inport  Port=5
  x|x|^2 : Inport  Port=6
  abs_x_4th_acc : Subsystem
  abs_x_sq_acc : Subsystem
  acc_rst : Subsystem
  x_acc : Subsystem
  x_cube_acc : Subsystem
  x_sq_acc : Subsystem
  sync_out : Outport
  "Re{E[x]}" : Outport  Port=2
  "Im{E[x]}" : Outport  Port=3
  "Re{E[x^2]}" : Outport  Port=4
  "Im{E[x^2]}" : Outport  Port=5
  E[|x|^2] : Outport  Port=6
  E[|x|^4] : Outport  Port=7
  "Re{E[x|x|^2]}" : Outport  Port=8
  "Im{E[x|x|^2]}" : Outport  Port=9
  wires:
  acc_rst/1(acc_rst) -> abs_x_4th_acc/1(sync), abs_x_sq_acc/1(sync), x_cube_acc/1(sync), x_sq_acc/1(sync), x_acc/1(sync)  "acc_rst"
  abs_x_4th_acc/1(+=b) -> E[|x|^4]/1
  |x|^4/1 -> abs_x_4th_acc/2(b)
  abs_x_sq_acc/1(+=b) -> E[|x|^2]/1
  |x|^2/1 -> abs_x_sq_acc/2(b)
  x_cube_acc/2(x_im_acc) -> "Im{E[x|x|^2]}"/1
  x_cube_acc/1(x_re_acc) -> "Re{E[x|x|^2]}"/1
  x|x|^2/1 -> x_cube_acc/2(x)
  x_sq_acc/2(x_im_acc) -> "Im{E[x^2]}"/1
  x_sq_acc/1(x_re_acc) -> "Re{E[x^2]}"/1
  x^2/1 -> x_sq_acc/2(x)
  x_acc/2(x_im_acc) -> "Im{E[x]}"/1
  x_acc/1(x_re_acc) -> "Re{E[x]}"/1
  x/1 -> x_acc/2(x)
  acc_rst/2(sync_out) -> sync_out/1
  sync/1 -> acc_rst/1(sync)

== system kurtosis/kurtosis/kurtosis_acc_bank_7 ==
  sync : Inport
  x : Inport  Port=2
  x^2 : Inport  Port=3
  |x|^2 : Inport  Port=4
  |x|^4 : Inport  Port=5
  x|x|^2 : Inport  Port=6
  abs_x_4th_acc : Subsystem
  abs_x_sq_acc : Subsystem
  acc_rst : Subsystem
  x_acc : Subsystem
  x_cube_acc : Subsystem
  x_sq_acc : Subsystem
  sync_out : Outport
  "Re{E[x]}" : Outport  Port=2
  "Im{E[x]}" : Outport  Port=3
  "Re{E[x^2]}" : Outport  Port=4
  "Im{E[x^2]}" : Outport  Port=5
  E[|x|^2] : Outport  Port=6
  E[|x|^4] : Outport  Port=7
  "Re{E[x|x|^2]}" : Outport  Port=8
  "Im{E[x|x|^2]}" : Outport  Port=9
  wires:
  acc_rst/1(acc_rst) -> abs_x_4th_acc/1(sync), abs_x_sq_acc/1(sync), x_cube_acc/1(sync), x_sq_acc/1(sync), x_acc/1(sync)  "acc_rst"
  abs_x_4th_acc/1(+=b) -> E[|x|^4]/1
  |x|^4/1 -> abs_x_4th_acc/2(b)
  abs_x_sq_acc/1(+=b) -> E[|x|^2]/1
  |x|^2/1 -> abs_x_sq_acc/2(b)
  x_cube_acc/2(x_im_acc) -> "Im{E[x|x|^2]}"/1
  x_cube_acc/1(x_re_acc) -> "Re{E[x|x|^2]}"/1
  x|x|^2/1 -> x_cube_acc/2(x)
  x_sq_acc/2(x_im_acc) -> "Im{E[x^2]}"/1
  x_sq_acc/1(x_re_acc) -> "Re{E[x^2]}"/1
  x^2/1 -> x_sq_acc/2(x)
  x_acc/2(x_im_acc) -> "Im{E[x]}"/1
  x_acc/1(x_re_acc) -> "Re{E[x]}"/1
  x/1 -> x_acc/2(x)
  acc_rst/2(sync_out) -> sync_out/1
  sync/1 -> acc_rst/1(sync)

== system kurtosis/kurtosis/kurtosis_acc_bank_8 ==
  sync : Inport
  x : Inport  Port=2
  x^2 : Inport  Port=3
  |x|^2 : Inport  Port=4
  |x|^4 : Inport  Port=5
  x|x|^2 : Inport  Port=6
  abs_x_4th_acc : Subsystem
  abs_x_sq_acc : Subsystem
  acc_rst : Subsystem
  x_acc : Subsystem
  x_cube_acc : Subsystem
  x_sq_acc : Subsystem
  sync_out : Outport
  "Re{E[x]}" : Outport  Port=2
  "Im{E[x]}" : Outport  Port=3
  "Re{E[x^2]}" : Outport  Port=4
  "Im{E[x^2]}" : Outport  Port=5
  E[|x|^2] : Outport  Port=6
  E[|x|^4] : Outport  Port=7
  "Re{E[x|x|^2]}" : Outport  Port=8
  "Im{E[x|x|^2]}" : Outport  Port=9
  wires:
  acc_rst/1(acc_rst) -> abs_x_4th_acc/1(sync), abs_x_sq_acc/1(sync), x_cube_acc/1(sync), x_sq_acc/1(sync), x_acc/1(sync)  "acc_rst"
  abs_x_4th_acc/1(+=b) -> E[|x|^4]/1
  |x|^4/1 -> abs_x_4th_acc/2(b)
  abs_x_sq_acc/1(+=b) -> E[|x|^2]/1
  |x|^2/1 -> abs_x_sq_acc/2(b)
  x_cube_acc/2(x_im_acc) -> "Im{E[x|x|^2]}"/1
  x_cube_acc/1(x_re_acc) -> "Re{E[x|x|^2]}"/1
  x|x|^2/1 -> x_cube_acc/2(x)
  x_sq_acc/2(x_im_acc) -> "Im{E[x^2]}"/1
  x_sq_acc/1(x_re_acc) -> "Re{E[x^2]}"/1
  x^2/1 -> x_sq_acc/2(x)
  x_acc/2(x_im_acc) -> "Im{E[x]}"/1
  x_acc/1(x_re_acc) -> "Re{E[x]}"/1
  x/1 -> x_acc/2(x)
  acc_rst/2(sync_out) -> sync_out/1
  sync/1 -> acc_rst/1(sync)

== system kurtosis/kurtosis/kurtosis_central_moment_calc ==
  sync : Inport
  channel_in : Inport  Port=2
  "Re{E[X]}" : Inport  Port=3
  "Im{E[X]}" : Inport  Port=4
  "Re{E[X^2]}" : Inport  Port=5
  "Im{E[X^2]}" : Inport  Port=6
  E[|X|^2] : Inport  Port=7
  E[||X||^4] : Inport  Port=8
  "Re{E[|X|^2X]}" : Inport  Port=9
  "Im{E[|X|^2X]}" : Inport  Port=10
  adder_tree_del : xbsIndex_r4/Convert  gui_display_data_type=Fixed-point  arith_type="Signed  (2's comp)"  n_bits=32  bin_pt=19  float_type=Single  exp_bits=8  fraction_bits=24  quantization="Round  (unbiased: +/- Inf)"  overflow=Saturate  en=off  latency=13  dbl_ovrd=off  pipeline=off  block_type=convert
  channel_del : xbsIndex_r4/Delay  rst=off  infoeditControl=Selection of Reset will increase slice count due to use of real FFs and instead of SRLs  en=off  latency=28  dbl_ovrd=off  reg_retiming=off  block_type=delay
  cross_product_del : xbsIndex_r4/Delay  rst=off  infoeditControl=Selection of Reset will increase slice count due to use of real FFs and instead of SRLs  en=off  latency=15  dbl_ovrd=off  reg_retiming=off  block_type=delay
  kurtosis_cross_products : Subsystem
  kurtosis_den : Subsystem
  kurtosis_num : Subsystem
  scale : xbsIndex_r4/Scale  scale_factor=-10  dbl_ovrd=off  block_type=scale
  sync_out : Outport
  channel : Outport  Port=2
  num : Outport  Port=3
  den : Outport  Port=4
  power : Outport  Port=5
  wires:
  E[|X|^2]/1 -> kurtosis_cross_products/6(E[|X|^2]), cross_product_del/1
  cross_product_del/1 -> kurtosis_den/1(E[|X|^2]), adder_tree_del/1
  channel_del/1 -> channel/1
  channel_in/1 -> channel_del/1
  kurtosis_num/2(E[|X-m_x|^4]) -> num/1
  kurtosis_num/1(sync_out) -> sync_out/1
  kurtosis_cross_products/9(|E[(x-mx)^2]|^2) -> kurtosis_num/8(|E[(x-mx)^2]|^2)
  kurtosis_cross_products/8(|m_x|^4) -> kurtosis_num/7(|m_x|^4)
  kurtosis_cross_products/6("Re{4E[X|X|^2*m_x]}") -> kurtosis_num/6("Re{4E[X|X|^2*m_x]}")
  kurtosis_cross_products/5("Re{2E[X^2*conj(m_x^2)]}") -> kurtosis_num/5("Re{2E[X^2*conj(m_x^2)]}")
  kurtosis_cross_products/4(E[|X|^4]) -> kurtosis_num/4(E[|X|^4])
  kurtosis_cross_products/3(4|m_x|^4) -> kurtosis_num/3(4|m_x|^4)
  kurtosis_cross_products/2(4E[|X|^2]|m_x|^2) -> kurtosis_num/2(4E[|X|^2]|m_x|^2)
  kurtosis_cross_products/1(sync_out) -> kurtosis_num/1(sync)
  kurtosis_den/1(E[|X-m_x|^2]^2) -> den/1
  kurtosis_cross_products/7(|m_x|^2) -> kurtosis_den/2(|m_x|^2)
  "Im{E[|X|^2X]}"/1 -> kurtosis_cross_products/9("Im{E[|X|^2X]}")
  "Re{E[|X|^2X]}"/1 -> kurtosis_cross_products/8("Re{E[|X|^2X]}")
  E[||X||^4]/1 -> kurtosis_cross_products/7(E[||X||^4])
  "Im{E[X^2]}"/1 -> kurtosis_cross_products/5("Im{E[X^2]}")
  "Re{E[X^2]}"/1 -> kurtosis_cross_products/4("Re{E[X^2]}")
  "Im{E[X]}"/1 -> kurtosis_cross_products/3("Im{E[X]}")
  "Re{E[X]}"/1 -> kurtosis_cross_products/2("Re{E[X]}")
  sync/1 -> kurtosis_cross_products/1(sync)
  scale/1 -> power/1
  adder_tree_del/1 -> scale/1

== system kurtosis/kurtosis/kurtosis_origin_moments_1 ==
  sync_in : Inport
  x_in : Inport  Port=2
  abs_x_sq : Subsystem
  abs_x_sq_del : xbsIndex_r4/Delay  rst=off  infoeditControl=Selection of Reset will increase slice count due to use of real FFs and instead of SRLs  en=off  latency=5  dbl_ovrd=off  reg_retiming=off  block_type=delay
  c_to_ri_xin : Subsystem
  cplx_sq : Subsystem
  ri_to_c_x_3rd : Subsystem
  square_real : xbsIndex_r4/Mult  precision=Full  arith_type="Signed  (2's comp)"  n_bits=36  bin_pt=34  quantization=Truncate  overflow=Wrap  en=off  latency=5  dbl_ovrd=off  use_behavioral_HDL=off  opt=Speed  use_embedded=on  optimum_pipeline=off  pipeline=on  use_rpm=on  placement_style=Triangular  block_type=mult
  sync_delay : xbsIndex_r4/Delay  rst=off  infoeditControl=Selection of Reset will increase slice count due to use of real FFs and instead of SRLs  en=off  latency=10  dbl_ovrd=off  reg_retiming=off  block_type=delay
  third_power_im : xbsIndex_r4/Mult  precision=Full  arith_type="Signed  (2's comp)"  n_bits=36  bin_pt=34  quantization=Truncate  overflow=Wrap  en=off  latency=5  dbl_ovrd=off  use_behavioral_HDL=off  opt=Speed  use_embedded=on  optimum_pipeline=off  pipeline=on  use_rpm=on  placement_style=Triangular  block_type=mult
  third_power_re : xbsIndex_r4/Mult  precision=Full  arith_type="Signed  (2's comp)"  n_bits=36  bin_pt=34  quantization=Truncate  overflow=Wrap  en=off  latency=5  dbl_ovrd=off  use_behavioral_HDL=off  opt=Speed  use_embedded=on  optimum_pipeline=off  pipeline=on  use_rpm=on  placement_style=Triangular  block_type=mult
  x_delay : xbsIndex_r4/Delay  rst=off  infoeditControl=Selection of Reset will increase slice count due to use of real FFs and instead of SRLs  en=off  latency=10  dbl_ovrd=off  reg_retiming=off  block_type=delay
  x_im_del : xbsIndex_r4/Delay  rst=off  infoeditControl=Selection of Reset will increase slice count due to use of real FFs and instead of SRLs  en=off  latency=5  dbl_ovrd=off  reg_retiming=off  block_type=delay
  x_re_del : xbsIndex_r4/Delay  rst=off  infoeditControl=Selection of Reset will increase slice count due to use of real FFs and instead of SRLs  en=off  latency=5  dbl_ovrd=off  reg_retiming=off  block_type=delay
  x_sq_del : xbsIndex_r4/Delay  rst=off  infoeditControl=Selection of Reset will increase slice count due to use of real FFs and instead of SRLs  en=off  latency=4  dbl_ovrd=off  reg_retiming=off  block_type=delay
  sync_out : Outport
  x : Outport  Port=2
  x^2 : Outport  Port=3
  |x|^2 : Outport  Port=4
  |x|^4 : Outport  Port=5
  x|x|^2 : Outport  Port=6
  wires:
  x_in/1 -> c_to_ri_xin/1(c), abs_x_sq/1(c), cplx_sq/2(b), cplx_sq/1(a), x_delay/1
  abs_x_sq/1(power) -> third_power_im/2, third_power_re/2, square_real/2, square_real/1, abs_x_sq_del/1
  ri_to_c_x_3rd/1(c) -> x|x|^2/1
  third_power_im/1 -> ri_to_c_x_3rd/2(im)
  third_power_re/1 -> ri_to_c_x_3rd/1(re)
  x_im_del/1 -> third_power_im/1
  x_re_del/1 -> third_power_re/1
  c_to_ri_xin/2(im) -> x_im_del/1
  c_to_ri_xin/1(re) -> x_re_del/1
  square_real/1 -> |x|^4/1
  abs_x_sq_del/1 -> |x|^2/1
  x_sq_del/1 -> x^2/1
  cplx_sq/1(c) -> x_sq_del/1
  x_delay/1 -> x/1
  sync_delay/1 -> sync_out/1
  sync_in/1 -> sync_delay/1
